simulink model "Commande"  (R2020b)
settings: Solver=VariableStepAuto  StartTime=0.0  StopTime=1  RelTol=1e-3
undefined symbols (not defined in the file or in its folder): FC, FuelCellLoadFcn, gcbh, ln, sps_rtmsupport, Ts
libraries: simulink x43, powerlib x37, powerlib_meascontrol x7, fuzblock x4, powerlib_extras x2
(part 1 of 3)
settings Model: Creator=Abdelhak_Samir  LastModifiedBy=Abdelhak_Samir
settings SolverCC: ZeroCrossAlgorithm=Adaptive
settings DebuggingCC: IgnoredZcDiagnostic=none  UnconnectedInputMsg=none  UnconnectedOutputMsg=none  UnconnectedLineMsg=none
settings ModelReferenceCC: EnableRefExpFcnMdlSchedulingChecks=off
settings RTWCC: GPUComputeCapability=5.0
settings ConfigComp: CovBoundaryAbsTol=1.0e-5

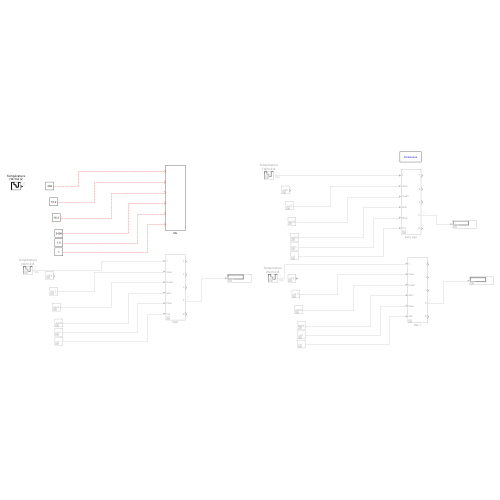
[thumbnail: Simulink's stored preview of the top-level diagram]
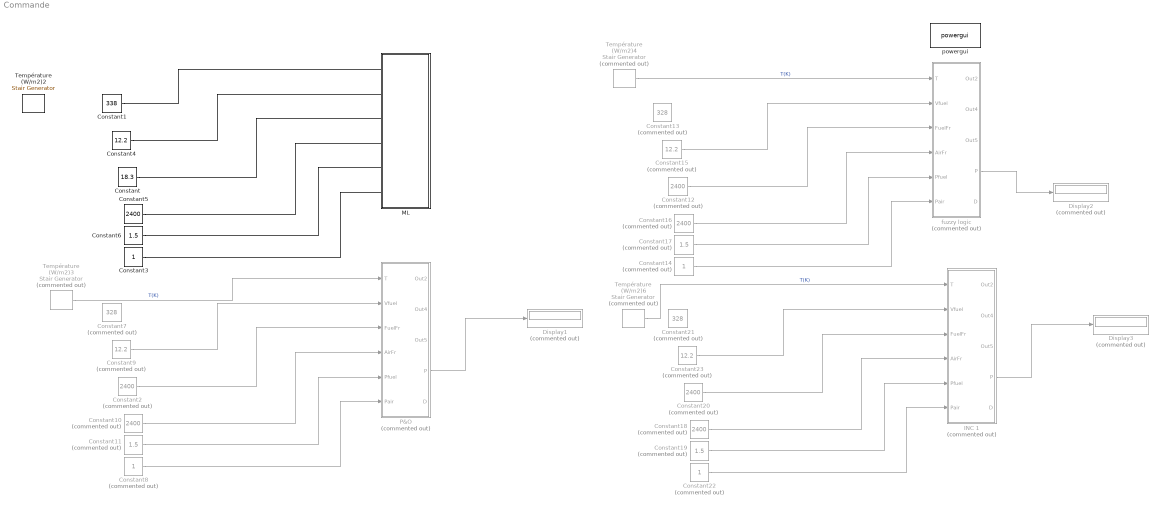
== system Commande ==
  Constant : Constant  Value=18.3
  Constant1 : Constant  Value=338
  Constant{2,10,12,16,18,20} (6 alike) : Constant  Commented=on  Value=2400
  Constant11 : Constant  Commented=on  Value=1.5
  Constant13 : Constant  Commented=on  Value=328
  Constant14 : Constant  Commented=on
  Constant15 : Constant  Commented=on  Value=12.2
  Constant17 : Constant  Commented=on  Value=1.5
  Constant19 : Constant  Commented=on  Value=1.5
  Constant21 : Constant  Commented=on  Value=328
  Constant22 : Constant  Commented=on
  Constant23 : Constant  Commented=on  Value=12.2
  Constant3 : Constant
  Constant4 : Constant  Value=12.2
  Constant5 : Constant  Value=2400
  Constant6 : Constant  Value=1.5
  Constant7 : Constant  Commented=on  Value=328
  Constant8 : Constant  Commented=on
  Constant9 : Constant  Commented=on  Value=12.2
  Display1 : Display  Commented=on
  Display2 : Display  Commented=on
  Display3 : Display  Commented=on
  INC 1 : Subsystem  Commented=on
  ML : Subsystem
  P&O : Subsystem  Commented=on
  Température (W/m2)2 : powerlib_meascontrol/Pulse & Signal Generators/Stair Generator  t=[0, 0.2 , 0.4 , 0.6, 0.8,1]  e=[300,330,320,310,330,330]  Ts=0.00001
  Température (W/m2)3 : powerlib_meascontrol/Pulse & Signal Generators/Stair Generator  Commented=on  t=[0, 0.2 , 0.4 , 0.6, 0.8,1]  e=[300,330,320,310,330,330]  Ts=0.00001
  Température (W/m2)4 : powerlib_meascontrol/Pulse & Signal Generators/Stair Generator  Commented=on  t=[0, 0.2 , 0.4 , 0.6, 0.8,1]  e=[300,330,320,310,330,330]  Ts=0.00001
  Température (W/m2)6 : powerlib_meascontrol/Pulse & Signal Generators/Stair Generator  Commented=on  t=[0, 0.2 , 0.4 , 0.6, 0.8,1]  e=[300,330,320,310,330,330]  Ts=0.00001
  fuzzy logic : Subsystem  Commented=on
  powergui : powerlib/powergui  Priority=1  SimulationMode=Continuous  SampleTime=0.0001  frequency=60  Iterations=50  frequencyindice=0  Pbase=100e6  ErrMax=1e-4  UnitsV=kV  UnitsW=MW  buscounter=0  FunctionMessages=off  echomessages=off  EnableUseOfTLC=off  CurrentSourceSwitches=off  DisableSnubberDevices=off  DisableRonSwitches=off  DisableVfSwitches=off  DisplayEquations=off  AutomaticDiscreteSolvers=off  SolverType=Tustin/Backward Euler (TBE)  Interpol=off  ExternalGateDelay=off  methode=off  Ts=100  x0status=blocks  SPID=on  SwTol=0  HookPort=off  NonlinearTolerance=1e-4  nMaxIteration=100  ContinueOnMaxIteration=off  RestoreLinks=warning  ResistiveCurrentMeasurement=off  Frange=[0:2:500]  Ylog=off  Xlog=on  ShowGrid=off  save=off  variable=ZData  structure=0  ZoomFFT=off  StartTime=0.0  cycles=1  DisplayStyle=1  fundamental=60  FreqAxis=off  MaxFrequency=1000  frequencyindicesteady=1  RmsSteady=1  display=off
  wires:
  Constant4/1 -> ?
  Constant/1 -> ?
  Constant5/1 -> ?
  Constant6/1 -> ?
  Constant3/1 -> ?
  Constant8/1 -> P&O/6(Pair)
  Constant2/1 -> P&O/3(FuelFr)
  Constant9/1 -> P&O/2(Vfuel)
  Constant10/1 -> P&O/4(AirFr)
  P&O/4(P) -> Display1/1
  Constant11/1 -> P&O/5(Pfuel)
  Constant14/1 -> fuzzy logic/6(Pair)
  Constant12/1 -> fuzzy logic/3(FuelFr)
  Constant15/1 -> fuzzy logic/2(Vfuel)
  Constant16/1 -> fuzzy logic/4(AirFr)
  fuzzy logic/4(P) -> Display2/1
  Constant17/1 -> fuzzy logic/5(Pfuel)
  INC 1/4(P) -> Display3/1
  Constant18/1 -> INC 1/4(AirFr)
  Constant20/1 -> INC 1/3(FuelFr)
  Constant22/1 -> INC 1/6(Pair)
  Constant23/1 -> INC 1/2(Vfuel)
  Constant19/1 -> INC 1/5(Pfuel)
  Température (W/m2)4/1 -> fuzzy logic/1(T)  "T(K)"
  Température (W/m2)3/1 -> P&O/1(T)  "T(K)"
  Température (W/m2)6/1 -> INC 1/1(T)  "T(K)"
  Constant1/1 -> ?

== system Commande/INC 1 ==
  note: LOAD
  note: Boost Convertor
  note: Voltage Sensor
  T : Inport
  Vfuel : Inport  Port=2
  FuelFr : Inport  Port=3
  AirFr : Inport  Port=4
  Pfuel : Inport  Port=5
  Pair : Inport  Port=6
  Current Measurement : powerlib/Measurements/Current Measurement  PhasorSimulation=off  OutputType=Complex  PSBequivalent=0
  Demux : Demux  Outputs=5
  Diode : powerlib/Power Electronics/Diode  Ron=0.001  Lon=0  Vf=0.7  IC=0  UseSnubber=0  Rs=500  Cs=250e-9  Measurements=off
  Diode1 : powerlib/Power Electronics/Diode  Ron=0.001  Lon=0  Vf=0.7  IC=0  UseSnubber=0  Rs=500  Cs=250e-9  Measurements=off
  E1 : Product  Inputs=**
  Fuel Cell Stack : Subsystem  AncestorBlock=sps_lib/Sources/Fuel Cell Stack  DialogController=POWERSYS.PowerSysDialog  LoadFcn=sps_rtmsupport('LoadFcn',gcbh);FuelCellLoadFcn(gcb)  StartFcn=sps_rtmsupport('StartFcn',gcbh);  StopFcn=sps_rtmsupport('StopFcn',gcbh);  mask(Fuel Cell Stack){PresetModel=PEMFC - 1.26 kW - 24 Vdc, FcType=0, Detailed=Detailed, Eoc=[42,35], NomVI=[52,24.23], EndVI=[100,20], Nc=42, n=46, TOp=55, AirFr=2400, SuppPress=[1.5,1], Comp=[99.95,21,1], SignX=off, SignY=off, FlowRateH2=on, FlowRateAir=on, SystemTemp=on, SystemPH2=off, SystemPAir=off, FCDyn=off, FC_tau=1, Peak_O2=80, V_Under=10}
      mask prompts: PresetModel "Preset model:"; FcType "Fuel Cell type:"; Detailed "Model detail Level:"; Eoc "Voltage at 0A and 1A [V_0(V), V_1(V)]"; NomVI "Nominal operating point [Inom(A), Vnom(V)]"; EndVI "Maximum operating point [Iend(A), Vend(V)]"; Nc "Number of cells"; n "Nominal stack efficiency (%)"; TOp "Operating temperature (Celsius)"; AirFr "Nominal Air flow rate (lpm)"; SuppPress "Nominal supply pressure [Fuel (bar), Air (bar)]"; Comp "Nominal composition (%) [H2 O2 H2O(Air)]"; SignX "Fuel  composition [x_H2(%)]"; SignY "Oxidant composition [y_O2(%)]"; FlowRateH2 "Fuel flow rate [FuelFr(lpm)]"; FlowRateAir "Air flow rate [AirFr(lpm)]"; SystemTemp "System Temperature [T(Kelvin)]"; SystemPH2 "Fuel supply pressure [Pfuel(bar)]"; SystemPAir "Air supply pressure [PAir(bar)]"; FCDyn "Specify Fuel Cell Dynamics?"; FC_tau "Fuel Cell response time (sec)"; Peak_O2 "Peak O2 utilization (%)"; V_Under "Voltage undershoot (V) @ peak O2 utilization"
      mask help:
      | Implements a generic hydrogen fuel cell model which allows the simulation for the following types of cells:
      | - Proton Exchange Membrane Fuel Cell (PEMFC)
      | - Solid Oxide Fuel Cell (SOFC)
      | - Alkaline Fuel Cell (AFC)
      mask init:
      | block = gcb;
      | %% DO NOT CHANGE THIS ORDER
      | FuelCellCback(block,'Inputs')
      | [FC, WantBlockChoice, Ts] = FuelCellInit(block,Eoc,NomVI,EndVI,Nc,n,TOp,AirFr,SuppPress,Comp,FlowRateH2,FlowRateAir);
      | powericon('SetInternalModels','set',block,WantBlockChoice);
      settings: CopyFcn=sps_rtmsupport('CopyFcn',gcbh);  DeleteFcn=sps_rtmsupport('DeleteFcn',gcbh);  UndoDeleteFcn=sps_rtmsupport('UndoDeleteFcn',gcbh);  ModelCloseFcn=sps_rtmsupport('ModelCloseFcn',gcbh);  PreSaveFcn=sps_rtmsupport('PreSaveFcn',gcbh);  PostSaveFcn=sps_rtmsupport('PostSaveFcn',gcbh);  NameChangeFcn=sps_rtmsupport('NameChangeFcn',gcbh);  PreCopyFcn=sps_rtmsupport('PreCopyFcn',gcbh);  OpenFcn=sps_rtmsupport('OpenFcn',gcbh, [1 2 3 13 14 15 16 17 18 19 20]);  CloseFcn=sps_rtmsupport('CloseFcn',gcbh);  PreDeleteFcn=sps_rtmsupport('PreDeleteFcn',gcbh);
      mask Help: helpview(psbhelp)
      mask TypeOptions PresetModel: No (User-Defined) | PEMFC - 1.26 kW - 24 Vdc | PEMFC - 6 kW - 45 Vdc | PEMFC - 50 kW - 625 Vdc | AFC - 2.4 kW - 48 Vdc | SOFC - 3 kW - 100 Vdc | SOFC - 25 kW - 630 Vdc
      mask Callback PresetModel: FuelCellCback(gcb,'Preset')
      mask TypeOptions Detailed: Simplified | Detailed
      mask Callback Detailed: FuelCellCback(gcb,'Visibilities')
      mask Callback FlowRateAir: FuelCellCback(gcb,'Visibilities')
      mask Callback FCDyn: FuelCellCback(gcb,'Visibilities')
      mask DialogControl ParameterTabVar0 Prompt: Parameters
      mask DialogControl plot_graph Prompt: Plot V_I characteristic
      mask DialogControl plot_graph Callback: FuelCellCback(gcb,'PlotGraph');
      mask DialogControl ViewParam Prompt: View Cell parameters
      mask DialogControl ViewParam Callback: FuelCellCback(gcb,'ViewParam');
      mask DialogControl ParameterTabVar01 Prompt: Signal variation
      mask DialogControl ParameterTabVar012 Prompt: Fuel Cell Dynamics
  Fuzzy Controller : Subsystem  Commented=on
  INC based MPPT : Subsystem
  Mosfet : powerlib/Power Electronics/Mosfet  Ron=0.1  Lon=0  Rd=0.01  Vfd=0.7  IC=0  Rs=1e5  Cs=10^-9  Measurements=off
  PWM Generator (DC-DC)1 : powerlib_meascontrol/Pulse & Signal Generators/PWM Generator (DC-DC)  Fsw=10000  Ts=0
  Pn : Product
  Scope : Scope  NumInputPorts=2
  Scope1 : Scope
  Scope2 : Scope
  Series RLC Branch : powerlib/Elements/Series RLC Branch  LConnTagsString=__new0  RConnTagsString=__new0  BranchType=L  Resistance=1  Inductance=1e-4  SetiL0=off  InitialCurrent=0  Capacitance=1e-6  Setx0=off  InitialVoltage=0  Measurements=None
  Series RLC Branch1 : powerlib/Elements/Series RLC Branch  LConnTagsString=__new0  RConnTagsString=__new0  BranchType=C  Resistance=1  Inductance=1e-4  SetiL0=off  InitialCurrent=0  Capacitance=4700e-6  Setx0=off  InitialVoltage=0  Measurements=None
  Series RLC Branch4 : powerlib/Elements/Series RLC Branch  LConnTagsString=__new0  RConnTagsString=__new0  BranchType=C  Resistance=1  Inductance=1e-4  SetiL0=off  InitialCurrent=0  Capacitance=4700e-5  Setx0=on  InitialVoltage=42  Measurements=None
  Series RLC Load1 : powerlib/Elements/Series RLC Load  LConnTagsString=a  RConnTagsString=__new0  NominalVoltage=50  NominalFrequency=500  ActivePower=33  InductivePower=0  CapacitivePower=0  Setx0=off  InitialVoltage=0  SetiL0=off  InitialCurrent=0  Measurements=None  LoadType=constant Z
  Voltage Measurement1 : powerlib/Measurements/Voltage Measurement  PhasorSimulation=off  OutputType=Complex  PSBequivalent=0
  Out2 : Outport
  Out4 : Outport  Port=2
  Out5 : Outport  Port=3
  P : Outport  Port=4
  D : Outport  Port=5
  wires:
  Current Measurement/1 -> E1/1  "Iout"
  Pn/1 -> P/1, Scope/2, Fuzzy Controller/2(P), Scope1/1  "P"
  PWM Generator (DC-DC)1/1 -> Mosfet/1
  Demux/1 -> Fuzzy Controller/1(Vin), INC based MPPT/1(Vpv), Scope2/1, Pn/1  "Vin"
  Fuzzy Controller/1(D) -> D/1
  Demux/5 -> Out5/1
  Demux/2 -> INC based MPPT/2(Ipv), Pn/2  "Iin"
  FuelFr/1 -> Fuel Cell Stack/1(FuelFr)
  Fuel Cell Stack/1(m) -> Demux/1
  E1/1 -> Scope/1  "Pout"
  AirFr/1 -> Fuel Cell Stack/2(AirFr)
  Voltage Measurement1/1 -> E1/2  "Vout"
  INC based MPPT/1(PWM1) -> PWM Generator (DC-DC)1/1
  Demux/3 -> Out2/1
  Demux/4 -> Out4/1
  T/1 -> Fuel Cell Stack/3(T)
  connections:
  Series RLC Branch4/LConn1 -- Series RLC Branch/LConn1 -- Diode1/RConn1
  Series RLC Branch1/LConn1 -- Diode/RConn1 -- Current Measurement/LConn1
  Fuel Cell Stack/RConn1 -- Diode1/LConn1
  Mosfet/RConn1 -- Fuel Cell Stack/RConn2 -- Series RLC Branch4/RConn1 -- Voltage Measurement1/LConn2 -- Series RLC Load1/RConn1 -- Series RLC Branch1/RConn1
  Current Measurement/RConn1 -- Series RLC Load1/LConn1 -- Voltage Measurement1/LConn1
  Mosfet/LConn1 -- Diode/LConn1 -- Series RLC Branch/RConn1

== system Commande/ML ==
  ML Model : Subsystem

== system Commande/P&O ==
  note: LOAD
  note: Boost Convertor
  note: Voltage Sensor
  T : Inport
  Vfuel : Inport  Port=2
  FuelFr : Inport  Port=3
  AirFr : Inport  Port=4
  Pfuel : Inport  Port=5
  Pair : Inport  Port=6
  Current Measurement : powerlib/Measurements/Current Measurement  PhasorSimulation=off  OutputType=Complex  PSBequivalent=0
  Demux : Demux  Outputs=5
  Diode : powerlib/Power Electronics/Diode  Ron=0.001  Lon=0  Vf=0.7  IC=0  UseSnubber=0  Rs=500  Cs=250e-9  Measurements=off
  Diode1 : powerlib/Power Electronics/Diode  Ron=0.001  Lon=0  Vf=0.7  IC=0  UseSnubber=0  Rs=500  Cs=250e-9  Measurements=off
  E1 : Product  Inputs=**
  Fuel Cell Stack : Subsystem  AncestorBlock=sps_lib/Sources/Fuel Cell Stack  DialogController=POWERSYS.PowerSysDialog  LoadFcn=sps_rtmsupport('LoadFcn',gcbh);FuelCellLoadFcn(gcb)  StartFcn=sps_rtmsupport('StartFcn',gcbh);  StopFcn=sps_rtmsupport('StopFcn',gcbh);  mask(Fuel Cell Stack){PresetModel=PEMFC - 1.26 kW - 24 Vdc, FcType=0, Detailed=Detailed, Eoc=[42,35], NomVI=[52,24.23], EndVI=[100,20], Nc=42, n=46, TOp=55, AirFr=2400, SuppPress=[1.5,1], Comp=[99.95,21,1], SignX=off, SignY=off, FlowRateH2=on, FlowRateAir=on, SystemTemp=on, SystemPH2=off, SystemPAir=off, FCDyn=off, FC_tau=1, Peak_O2=80, V_Under=10}
      mask prompts: PresetModel "Preset model:"; FcType "Fuel Cell type:"; Detailed "Model detail Level:"; Eoc "Voltage at 0A and 1A [V_0(V), V_1(V)]"; NomVI "Nominal operating point [Inom(A), Vnom(V)]"; EndVI "Maximum operating point [Iend(A), Vend(V)]"; Nc "Number of cells"; n "Nominal stack efficiency (%)"; TOp "Operating temperature (Celsius)"; AirFr "Nominal Air flow rate (lpm)"; SuppPress "Nominal supply pressure [Fuel (bar), Air (bar)]"; Comp "Nominal composition (%) [H2 O2 H2O(Air)]"; SignX "Fuel  composition [x_H2(%)]"; SignY "Oxidant composition [y_O2(%)]"; FlowRateH2 "Fuel flow rate [FuelFr(lpm)]"; FlowRateAir "Air flow rate [AirFr(lpm)]"; SystemTemp "System Temperature [T(Kelvin)]"; SystemPH2 "Fuel supply pressure [Pfuel(bar)]"; SystemPAir "Air supply pressure [PAir(bar)]"; FCDyn "Specify Fuel Cell Dynamics?"; FC_tau "Fuel Cell response time (sec)"; Peak_O2 "Peak O2 utilization (%)"; V_Under "Voltage undershoot (V) @ peak O2 utilization"
      mask help:
      | Implements a generic hydrogen fuel cell model which allows the simulation for the following types of cells:
      | - Proton Exchange Membrane Fuel Cell (PEMFC)
      | - Solid Oxide Fuel Cell (SOFC)
      | - Alkaline Fuel Cell (AFC)
      mask init: same as Commande/INC 1/Fuel Cell Stack
      settings: CopyFcn=sps_rtmsupport('CopyFcn',gcbh);  DeleteFcn=sps_rtmsupport('DeleteFcn',gcbh);  UndoDeleteFcn=sps_rtmsupport('UndoDeleteFcn',gcbh);  ModelCloseFcn=sps_rtmsupport('ModelCloseFcn',gcbh);  PreSaveFcn=sps_rtmsupport('PreSaveFcn',gcbh);  PostSaveFcn=sps_rtmsupport('PostSaveFcn',gcbh);  NameChangeFcn=sps_rtmsupport('NameChangeFcn',gcbh);  PreCopyFcn=sps_rtmsupport('PreCopyFcn',gcbh);  OpenFcn=sps_rtmsupport('OpenFcn',gcbh, [1 2 3 13 14 15 16 17 18 19 20]);  CloseFcn=sps_rtmsupport('CloseFcn',gcbh);  PreDeleteFcn=sps_rtmsupport('PreDeleteFcn',gcbh);
      mask Help: helpview(psbhelp)
      mask TypeOptions PresetModel: No (User-Defined) | PEMFC - 1.26 kW - 24 Vdc | PEMFC - 6 kW - 45 Vdc | PEMFC - 50 kW - 625 Vdc | AFC - 2.4 kW - 48 Vdc | SOFC - 3 kW - 100 Vdc | SOFC - 25 kW - 630 Vdc
      mask Callback PresetModel: FuelCellCback(gcb,'Preset')
      mask TypeOptions Detailed: Simplified | Detailed
      mask Callback Detailed: FuelCellCback(gcb,'Visibilities')
      mask Callback FlowRateAir: FuelCellCback(gcb,'Visibilities')
      mask Callback FCDyn: FuelCellCback(gcb,'Visibilities')
      mask DialogControl ParameterTabVar0 Prompt: Parameters
      mask DialogControl plot_graph Prompt: Plot V_I characteristic
      mask DialogControl plot_graph Callback: FuelCellCback(gcb,'PlotGraph');
      mask DialogControl ViewParam Prompt: View Cell parameters
      mask DialogControl ViewParam Callback: FuelCellCback(gcb,'ViewParam');
      mask DialogControl ParameterTabVar01 Prompt: Signal variation
      mask DialogControl ParameterTabVar012 Prompt: Fuel Cell Dynamics
  Fuzzy Controller : Subsystem  Commented=on
  Mosfet : powerlib/Power Electronics/Mosfet  Ron=0.1  Lon=0  Rd=0.01  Vfd=0.7  IC=0  Rs=1e5  Cs=10^-9  Measurements=off
  P&O base MPPT : Subsystem
  PWM Generator (DC-DC)1 : powerlib_meascontrol/Pulse & Signal Generators/PWM Generator (DC-DC)  Fsw=10000  Ts=0
  Pn : Product
  Scope : Scope  NumInputPorts=2
  Scope1 : Scope
  Scope2 : Scope
  Series RLC Branch : powerlib/Elements/Series RLC Branch  LConnTagsString=__new0  RConnTagsString=__new0  BranchType=L  Resistance=1  Inductance=1e-4  SetiL0=off  InitialCurrent=0  Capacitance=1e-6  Setx0=off  InitialVoltage=0  Measurements=None
  Series RLC Branch1 : powerlib/Elements/Series RLC Branch  LConnTagsString=__new0  RConnTagsString=__new0  BranchType=C  Resistance=1  Inductance=1e-4  SetiL0=off  InitialCurrent=0  Capacitance=4700e-6  Setx0=off  InitialVoltage=0  Measurements=None
  Series RLC Branch4 : powerlib/Elements/Series RLC Branch  LConnTagsString=__new0  RConnTagsString=__new0  BranchType=C  Resistance=1  Inductance=1e-4  SetiL0=off  InitialCurrent=0  Capacitance=4700e-5  Setx0=on  InitialVoltage=42  Measurements=None
  Series RLC Load1 : powerlib/Elements/Series RLC Load  LConnTagsString=a  RConnTagsString=__new0  NominalVoltage=50  NominalFrequency=500  ActivePower=33  InductivePower=0  CapacitivePower=0  Setx0=off  InitialVoltage=0  SetiL0=off  InitialCurrent=0  Measurements=None  LoadType=constant Z
  Voltage Measurement1 : powerlib/Measurements/Voltage Measurement  PhasorSimulation=off  OutputType=Complex  PSBequivalent=0
  Out2 : Outport
  Out4 : Outport  Port=2
  Out5 : Outport  Port=3
  P : Outport  Port=4
  D : Outport  Port=5
  wires:
  Current Measurement/1 -> E1/1  "Iout"
  Pn/1 -> P/1, Scope/2, Fuzzy Controller/2(P), Scope1/1  "P"
  PWM Generator (DC-DC)1/1 -> Mosfet/1
  Demux/1 -> Scope2/1, Fuzzy Controller/1(Vin), P&O base MPPT/1(Vpv), Pn/1  "Vin"
  Fuzzy Controller/1(D) -> D/1
  Demux/5 -> Out5/1
  Demux/2 -> P&O base MPPT/2(Ipv), Pn/2  "Iin"
  FuelFr/1 -> Fuel Cell Stack/1(FuelFr)
  Fuel Cell Stack/1(m) -> Demux/1
  E1/1 -> Scope/1  "Pout"
  AirFr/1 -> Fuel Cell Stack/2(AirFr)
  Voltage Measurement1/1 -> E1/2  "Vout"
  P&O base MPPT/1(PWM) -> PWM Generator (DC-DC)1/1
  Demux/3 -> Out2/1
  Demux/4 -> Out4/1
  T/1 -> Fuel Cell Stack/3(T)
  connections:
  Series RLC Branch4/LConn1 -- Series RLC Branch/LConn1 -- Diode1/RConn1
  Series RLC Branch1/LConn1 -- Diode/RConn1 -- Current Measurement/LConn1
  Fuel Cell Stack/RConn1 -- Diode1/LConn1
  Mosfet/RConn1 -- Fuel Cell Stack/RConn2 -- Series RLC Branch4/RConn1 -- Voltage Measurement1/LConn2 -- Series RLC Load1/RConn1 -- Series RLC Branch1/RConn1
  Current Measurement/RConn1 -- Series RLC Load1/LConn1 -- Voltage Measurement1/LConn1
  Mosfet/LConn1 -- Diode/LConn1 -- Series RLC Branch/RConn1

== system Commande/fuzzy logic ==
  note: LOAD
  note: Boost Convertor
  note: Voltage Sensor
  T : Inport
  Vfuel : Inport  Port=2
  FuelFr : Inport  Port=3
  AirFr : Inport  Port=4
  Pfuel : Inport  Port=5
  Pair : Inport  Port=6
  Constant : Constant  Value=330
  Current Measurement : powerlib/Measurements/Current Measurement  PhasorSimulation=off  OutputType=Complex  PSBequivalent=0
  Demux : Demux  Outputs=5
  Diode : powerlib/Power Electronics/Diode  Ron=0.001  Lon=0  Vf=0.7  IC=0  UseSnubber=0  Rs=500  Cs=250e-9  Measurements=off
  Diode1 : powerlib/Power Electronics/Diode  Ron=0.001  Lon=0  Vf=0.7  IC=0  UseSnubber=0  Rs=500  Cs=250e-9  Measurements=off
  Display : Display
  E1 : Product  Inputs=**
  Fuel Cell Stack1 : Subsystem  AncestorBlock=sps_lib/Sources/Fuel Cell Stack  DialogController=POWERSYS.PowerSysDialog  LoadFcn=sps_rtmsupport('LoadFcn',gcbh);FuelCellLoadFcn(gcb)  StartFcn=sps_rtmsupport('StartFcn',gcbh);  StopFcn=sps_rtmsupport('StopFcn',gcbh);  mask(Fuel Cell Stack){PresetModel=PEMFC - 1.26 kW - 24 Vdc, FcType=0, Detailed=Detailed, Eoc=[42,35], NomVI=[52,24.23], EndVI=[100,20], Nc=42, n=46, TOp=55, AirFr=2400, SuppPress=[1.5,1], Comp=[99.95,21,1], SignX=off, SignY=off, FlowRateH2=on, FlowRateAir=on, SystemTemp=on, SystemPH2=off, SystemPAir=off, FCDyn=off, FC_tau=1, Peak_O2=80, V_Under=10}
      mask prompts: PresetModel "Preset model:"; FcType "Fuel Cell type:"; Detailed "Model detail Level:"; Eoc "Voltage at 0A and 1A [V_0(V), V_1(V)]"; NomVI "Nominal operating point [Inom(A), Vnom(V)]"; EndVI "Maximum operating point [Iend(A), Vend(V)]"; Nc "Number of cells"; n "Nominal stack efficiency (%)"; TOp "Operating temperature (Celsius)"; AirFr "Nominal Air flow rate (lpm)"; SuppPress "Nominal supply pressure [Fuel (bar), Air (bar)]"; Comp "Nominal composition (%) [H2 O2 H2O(Air)]"; SignX "Fuel  composition [x_H2(%)]"; SignY "Oxidant composition [y_O2(%)]"; FlowRateH2 "Fuel flow rate [FuelFr(lpm)]"; FlowRateAir "Air flow rate [AirFr(lpm)]"; SystemTemp "System Temperature [T(Kelvin)]"; SystemPH2 "Fuel supply pressure [Pfuel(bar)]"; SystemPAir "Air supply pressure [PAir(bar)]"; FCDyn "Specify Fuel Cell Dynamics?"; FC_tau "Fuel Cell response time (sec)"; Peak_O2 "Peak O2 utilization (%)"; V_Under "Voltage undershoot (V) @ peak O2 utilization"
      mask help:
      | Implements a generic hydrogen fuel cell model which allows the simulation for the following types of cells:
      | - Proton Exchange Membrane Fuel Cell (PEMFC)
      | - Solid Oxide Fuel Cell (SOFC)
      | - Alkaline Fuel Cell (AFC)
      mask init: same as Commande/INC 1/Fuel Cell Stack
      settings: CopyFcn=sps_rtmsupport('CopyFcn',gcbh);  DeleteFcn=sps_rtmsupport('DeleteFcn',gcbh);  UndoDeleteFcn=sps_rtmsupport('UndoDeleteFcn',gcbh);  ModelCloseFcn=sps_rtmsupport('ModelCloseFcn',gcbh);  PreSaveFcn=sps_rtmsupport('PreSaveFcn',gcbh);  PostSaveFcn=sps_rtmsupport('PostSaveFcn',gcbh);  NameChangeFcn=sps_rtmsupport('NameChangeFcn',gcbh);  PreCopyFcn=sps_rtmsupport('PreCopyFcn',gcbh);  OpenFcn=sps_rtmsupport('OpenFcn',gcbh, [1 2 3 13 14 15 16 17 18 19 20]);  CloseFcn=sps_rtmsupport('CloseFcn',gcbh);  PreDeleteFcn=sps_rtmsupport('PreDeleteFcn',gcbh);
      mask Help: helpview(psbhelp)
      mask TypeOptions PresetModel: No (User-Defined) | PEMFC - 1.26 kW - 24 Vdc | PEMFC - 6 kW - 45 Vdc | PEMFC - 50 kW - 625 Vdc | AFC - 2.4 kW - 48 Vdc | SOFC - 3 kW - 100 Vdc | SOFC - 25 kW - 630 Vdc
      mask Callback PresetModel: FuelCellCback(gcb,'Preset')
      mask TypeOptions Detailed: Simplified | Detailed
      mask Callback Detailed: FuelCellCback(gcb,'Visibilities')
      mask Callback FlowRateAir: FuelCellCback(gcb,'Visibilities')
      mask Callback FCDyn: FuelCellCback(gcb,'Visibilities')
      mask DialogControl ParameterTabVar0 Prompt: Parameters
      mask DialogControl plot_graph Prompt: Plot V_I characteristic
      mask DialogControl plot_graph Callback: FuelCellCback(gcb,'PlotGraph');
      mask DialogControl ViewParam Prompt: View Cell parameters
      mask DialogControl ViewParam Callback: FuelCellCback(gcb,'ViewParam');
      mask DialogControl ParameterTabVar01 Prompt: Signal variation
      mask DialogControl ParameterTabVar012 Prompt: Fuel Cell Dynamics
  Fuzzy Controller : Subsystem  Commented=on
  Fuzzy Controller2 : Subsystem
  Mosfet : powerlib/Power Electronics/Mosfet  Ron=0.1  Lon=0  Rd=0.01  Vfd=0.7  IC=0  Rs=1e5  Cs=10^-9  Measurements=off
  PWM Generator (DC-DC) : powerlib_meascontrol/Pulse & Signal Generators/PWM Generator (DC-DC)  Fsw=10000  Ts=0
  Pn : Product
  Scope : Scope  NumInputPorts=2
  Series RLC Branch : powerlib/Elements/Series RLC Branch  LConnTagsString=__new0  RConnTagsString=__new0  BranchType=L  Resistance=1  Inductance=1e-4  SetiL0=off  InitialCurrent=0  Capacitance=1e-6  Setx0=off  InitialVoltage=0  Measurements=None
  Series RLC Branch1 : powerlib/Elements/Series RLC Branch  LConnTagsString=__new0  RConnTagsString=__new0  BranchType=C  Resistance=1  Inductance=1e-4  SetiL0=off  InitialCurrent=0  Capacitance=4700e-6  Setx0=off  InitialVoltage=0  Measurements=None
  Series RLC Branch4 : powerlib/Elements/Series RLC Branch  LConnTagsString=__new0  RConnTagsString=__new0  BranchType=C  Resistance=1  Inductance=1e-4  SetiL0=off  InitialCurrent=0  Capacitance=4700e-5  Setx0=on  InitialVoltage=42  Measurements=None
  Series RLC Load1 : powerlib/Elements/Series RLC Load  LConnTagsString=a  RConnTagsString=__new0  NominalVoltage=50  NominalFrequency=500  ActivePower=33  InductivePower=0  CapacitivePower=0  Setx0=off  InitialVoltage=0  SetiL0=off  InitialCurrent=0  Measurements=None  LoadType=constant Z
  Voltage Measurement1 : powerlib/Measurements/Voltage Measurement  PhasorSimulation=off  OutputType=Complex  PSBequivalent=0
  Out2 : Outport
  Out4 : Outport  Port=2
  Out5 : Outport  Port=3
  P : Outport  Port=4
  D : Outport  Port=5
  wires:
  Current Measurement/1 -> E1/1  "Iout"
  Pn/1 -> Fuzzy Controller2/2(P), Display/1, P/1, Scope/2, Fuzzy Controller/2(P)  "P"
  Demux/1 -> Fuzzy Controller2/1(Vin), Fuzzy Controller/1(Vin), Pn/1  "Vin"
  Fuzzy Controller/1(D) -> D/1
  Demux/5 -> Out5/1
  Demux/2 -> Pn/2  "Iin"
  Fuel Cell Stack1/1(m) -> Demux/1
  E1/1 -> Scope/1  "Pout"
  Voltage Measurement1/1 -> E1/2  "Vout"
  PWM Generator (DC-DC)/1 -> Mosfet/1
  Demux/3 -> Out2/1
  Demux/4 -> Out4/1
  Fuzzy Controller2/1(D) -> PWM Generator (DC-DC)/1
  AirFr/1 -> Fuel Cell Stack1/2(AirFr)
  FuelFr/1 -> Fuel Cell Stack1/1(FuelFr)
  T/1 -> Fuel Cell Stack1/3(T)
  connections:
  Series RLC Branch4/LConn1 -- Series RLC Branch/LConn1 -- Diode1/RConn1
  Series RLC Branch1/LConn1 -- Diode/RConn1 -- Current Measurement/LConn1
  Fuel Cell Stack1/RConn1 -- Diode1/LConn1
  Mosfet/RConn1 -- Fuel Cell Stack1/RConn2 -- Series RLC Branch4/RConn1 -- Series RLC Load1/RConn1 -- Voltage Measurement1/LConn2 -- Series RLC Branch1/RConn1
  Current Measurement/RConn1 -- Voltage Measurement1/LConn1 -- Series RLC Load1/LConn1
  Mosfet/LConn1 -- Diode/LConn1 -- Series RLC Branch/RConn1

== system Commande/INC 1/Fuel Cell Stack ==
  FuelFr : Inport
  AirFr : Inport  Port=2
  T : Inport  Port=3
  Controlled Voltage Source1 : powerlib/Electrical Sources/Controlled Voltage Source  Initialize=on  Source_Type=AC  Amplitude=0  Phase=0  Frequency=0  Measurements=None
  Current Measurement1 : powerlib/Measurements/Current Measurement  PhasorSimulation=off  OutputType=Complex  PSBequivalent=0
  Diode1 : powerlib/Power Electronics/Diode  Ron=FC.Rohm  Lon=0  Vf=0  IC=0  UseSnubber=off  Rs=1e4  Cs=inf  Measurements=off
  Gain1 : Gain  Gain=0.01
  Gain3 : Gain  Gain=0.01
  Model : Subsystem  AncestorBlock=sps_lib/Sources/Fuel Cell Stack/Model  Variant=on  VariantControlMode=label  LabelModeActiveChoice=Continuous/Detailed
      settings: AttributesFormatString=%<BlockChoice>
  PAir : Constant  Value=FC.PAir
  Pfuel : Constant  Value=FC.Pf
  x_H2 : Constant  Value=FC.x*100
  y_O2 : Constant  Value=FC.y*100
  + : PMIOPort  Tag=PMCPort  Side=Right
  - : PMIOPort  Tag=PMCPort  Port=2  Side=Right
  m : Outport  VectorParamsAs1DForOutWhenUnconnected=off
  wires:
  PAir/1 -> Model/8(PAir)
  Pfuel/1 -> Model/7(Pf)
  T/1 -> Model/2(Op Temp)
  Model/1(Voltage) -> Controlled Voltage Source1/1
  Current Measurement1/1 -> Model/1(Current)
  Model/2(m) -> m/1
  FuelFr/1 -> Model/3(H2)
  x_H2/1 -> Gain1/1
  AirFr/1 -> Model/5(Air)
  y_O2/1 -> Gain3/1
  Gain1/1 -> Model/4(x_H2)
  Gain3/1 -> Model/6(y_O2)
  connections:
  Current Measurement1/LConn1 -- Controlled Voltage Source1/RConn1
  Current Measurement1/RConn1 -- Diode1/LConn1
  -/RConn1 -- Controlled Voltage Source1/LConn1
  Diode1/RConn1 -- +/RConn1

== system Commande/INC 1/Fuzzy Controller ==
  note: DE
  Vin : Inport
  P : Inport  Port=2
  Add : Sum
  DE : Sum  Inputs=+-
  E : Product  Inputs=/*
  Fuzzy Logic Controller with Ruleviewer : fuzblock/Fuzzy Logic  Controller  with Ruleviewer  fismatrix=twnty_five_rules_2  Ts=0.1
  Gain1 : Gain
  Memory1 : Memory  InheritSampleTime=on
  Memory2 : Memory  InheritSampleTime=on
  Memory3 : Memory
  Memory4 : Memory  InheritSampleTime=on
  Mux : Mux  Inputs=2
  Saturation : Saturate  UpperLimit=0.9  LowerLimit=0.1
  Zero-Order Hold : ZeroOrderHold  SampleTime=-1
  Zero-Order Hold1 : ZeroOrderHold  SampleTime=-1
  dP : Sum  Inputs=|+-
  dV : Sum  Inputs=-+
  D : Outport
  wires:
  DE/1 -> Mux/2  "DE"
  Fuzzy Logic Controller with Ruleviewer/1 -> Gain1/1  "DeltaD_Pur"
  Zero-Order Hold/1 -> dP/2, Memory1/1
  dV/1 -> E/1
  dP/1 -> E/2
  E/1 -> DE/1, Memory2/1, Mux/1  "E"
  Mux/1 -> Fuzzy Logic Controller with Ruleviewer/1
  Memory4/1 -> dV/1
  Memory1/1 -> dP/1
  Zero-Order Hold1/1 -> Memory4/1, dV/2
  Gain1/1 -> Add/1  "DeltaD"
  Memory3/1 -> Add/2
  Saturation/1 -> D/1, Memory3/1  "D"
  Memory2/1 -> DE/2
  Add/1 -> Saturation/1
  Vin/1 -> Zero-Order Hold1/1
  P/1 -> Zero-Order Hold/1

== system Commande/INC 1/INC based MPPT ==
  Vpv : Inport
  Ipv : Inport  Port=2
  Add1 : Sum  Inputs=|++
  Add2 : Sum  Inputs=+-
  Add3 : Sum  Inputs=+-
  Add4 : Sum  Inputs=+-
  Compare To Zero : simulink/Logic and Bit Operations/Compare To Zero  relop=~=  OutDataTypeStr=uint8
  Constant2 : Constant  Value=1e-6
  Dead Zone1 : DeadZone  LowerValue=-0.02  UpperValue=+0.02  SaturateOnIntegerOverflow=on
  Gain : Gain
  Initial Duty Cycle1 : Constant  Value=0.5
  Saturation : Saturate  UpperLimit=0.9  LowerLimit=0.1
  Saturation1 : Saturate  UpperLimit=inf  LowerLimit=eps
  Switch2 : Switch  Criteria=u2 ~= 0
  Vb : Memory  InheritSampleTime=on  LinearizeAsDelay=on
  Vb1 : Memory  InheritSampleTime=on  LinearizeAsDelay=on
  div1 : Product  Inputs=*/  RndMeth=Zero
  div2 : Product  Inputs=*/  RndMeth=Zero
  PWM1 : Outport
  wires:
  Add4/1 -> Saturation/1  "D"
  Gain/1 -> Add4/2
  Initial Duty Cycle1/1 -> Add4/1
  Add3/1 -> Compare To Zero/1, Switch2/1  "dV"
  div2/1 -> Add1/2  "I/V"
  Saturation1/1 -> div2/2
  Vb1/1 -> Add3/2
  Add2/1 -> div1/1  "dI"
  Switch2/1 -> div1/2
  Vb/1 -> Add2/2
  Ipv/1 -> Vb/1, Add2/1, div2/1  "I"
  div1/1 -> Add1/1  "dI/dV"
  Compare To Zero/1 -> Switch2/2
  Constant2/1 -> Switch2/3
  Vpv/1 -> Add3/1, Vb1/1, Saturation1/1  "V"
  Add1/1 -> Gain/1  "error"
  Saturation/1 -> PWM1/1

== system Commande/ML/ML Model ==
  Vin : Inport
  T : Inport  Port=2
  Vfuel : Inport  Port=3
  Vout : Inport  Port=4
  Vair : Inport  Port=5
  Pfuel : Inport  Port=6
  Pair : Inport  Port=7
  Constant8 : Constant
  E : Product  Inputs=*/
  Gain : Gain  Gain=1000
  MATLAB Function : MATLAB Function  TreatAsAtomicUnit=on
  Saturation : Saturate  UpperLimit=0.9  LowerLimit=0.1
  Scope3 : Scope
  Sum1 : Sum  Inputs=|+-
  Sum2 : Sum  Inputs=|+-
  D : Outport
  wires:
  Saturation/1 -> D/1, Scope3/1
  Gain/1 -> E/1
  MATLAB Function/1(Vmpp) -> Sum2/1  "Vref"
  Sum1/1 -> Saturation/1  "D"
  Pair/1 -> MATLAB Function/3(Pair)
  Sum2/1 -> Gain/1  "D"
  E/1 -> Sum1/2
  T/1 -> MATLAB Function/1(T)
  Constant8/1 -> Sum1/1
  Vin/1 -> Sum2/2
  Vout/1 -> E/2
  Pfuel/1 -> MATLAB Function/2(Pfuel)
  Vfuel/1 -> MATLAB Function/4(Vfuel)
  Vair/1 -> MATLAB Function/5(Vair)

== system Commande/P&O/Fuel Cell Stack ==
  FuelFr : Inport
  AirFr : Inport  Port=2
  T : Inport  Port=3
  Controlled Voltage Source1 : powerlib/Electrical Sources/Controlled Voltage Source  Initialize=on  Source_Type=AC  Amplitude=0  Phase=0  Frequency=0  Measurements=None
  Current Measurement1 : powerlib/Measurements/Current Measurement  PhasorSimulation=off  OutputType=Complex  PSBequivalent=0
  Diode1 : powerlib/Power Electronics/Diode  Ron=FC.Rohm  Lon=0  Vf=0  IC=0  UseSnubber=off  Rs=1e4  Cs=inf  Measurements=off
  Gain1 : Gain  Gain=0.01
  Gain3 : Gain  Gain=0.01
  Model : Subsystem  AncestorBlock=sps_lib/Sources/Fuel Cell Stack/Model  Variant=on  VariantControlMode=label  LabelModeActiveChoice=Continuous/Detailed
      settings: AttributesFormatString=%<BlockChoice>
  PAir : Constant  Value=FC.PAir
  Pfuel : Constant  Value=FC.Pf
  x_H2 : Constant  Value=FC.x*100
  y_O2 : Constant  Value=FC.y*100
  + : PMIOPort  Tag=PMCPort  Side=Right
  - : PMIOPort  Tag=PMCPort  Port=2  Side=Right
  m : Outport  VectorParamsAs1DForOutWhenUnconnected=off
  wires:
  PAir/1 -> Model/8(PAir)
  Pfuel/1 -> Model/7(Pf)
  T/1 -> Model/2(Op Temp)
  Model/1(Voltage) -> Controlled Voltage Source1/1
  Current Measurement1/1 -> Model/1(Current)
  Model/2(m) -> m/1
  FuelFr/1 -> Model/3(H2)
  x_H2/1 -> Gain1/1
  AirFr/1 -> Model/5(Air)
  y_O2/1 -> Gain3/1
  Gain1/1 -> Model/4(x_H2)
  Gain3/1 -> Model/6(y_O2)
  connections:
  Current Measurement1/LConn1 -- Controlled Voltage Source1/RConn1
  Current Measurement1/RConn1 -- Diode1/LConn1
  -/RConn1 -- Controlled Voltage Source1/LConn1
  Diode1/RConn1 -- +/RConn1

== system Commande/P&O/Fuzzy Controller ==
  note: DE
  Vin : Inport
  P : Inport  Port=2
  Add : Sum
  DE : Sum  Inputs=+-
  E : Product  Inputs=/*
  Fuzzy Logic Controller with Ruleviewer : fuzblock/Fuzzy Logic  Controller  with Ruleviewer  fismatrix=twnty_five_rules_2  Ts=0.1
  Gain1 : Gain
  Memory1 : Memory  InheritSampleTime=on
  Memory2 : Memory  InheritSampleTime=on
  Memory3 : Memory
  Memory4 : Memory  InheritSampleTime=on
  Mux : Mux  Inputs=2
  Saturation : Saturate  UpperLimit=0.9  LowerLimit=0.1
  Zero-Order Hold : ZeroOrderHold  SampleTime=-1
  Zero-Order Hold1 : ZeroOrderHold  SampleTime=-1
  dP : Sum  Inputs=|+-
  dV : Sum  Inputs=-+
  D : Outport
  wires:
  DE/1 -> Mux/2  "DE"
  Fuzzy Logic Controller with Ruleviewer/1 -> Gain1/1  "DeltaD_Pur"
  Zero-Order Hold/1 -> dP/2, Memory1/1
  dV/1 -> E/1
  dP/1 -> E/2
  E/1 -> DE/1, Memory2/1, Mux/1  "E"
  Mux/1 -> Fuzzy Logic Controller with Ruleviewer/1
  Memory4/1 -> dV/1
  Memory1/1 -> dP/1
  Zero-Order Hold1/1 -> Memory4/1, dV/2
  Gain1/1 -> Add/1  "DeltaD"
  Memory3/1 -> Add/2
  Saturation/1 -> D/1, Memory3/1  "D"
  Memory2/1 -> DE/2
  Add/1 -> Saturation/1
  Vin/1 -> Zero-Order Hold1/1
  P/1 -> Zero-Order Hold/1

== system Commande/P&O/P&O base MPPT ==
  note: D
  Vpv : Inport
  Ipv : Inport  Port=2
  D State : Product  RndMeth=Zero
  DeltaD : Constant  Value=0.05
  DeltaP*DeltaV : Product  RndMeth=Zero
  I Filter : powerlib_extras/Control  Blocks/1st-Order  Filter  FilterType=Lowpass  Tc=1e-3  Initialize=off  Vac_Init=[0.8 -25 60]  Vdc_Init=-0.4  PlotResponse=off  param1=[1 500 1]
  Ib : Memory  InheritSampleTime=on  LinearizeAsDelay=on
  If DeltaP*DeltaV<0 : Constant
  If DeltaP*DeltaV>0 : Constant  Value=-1
  Memory2 : Memory  InheritSampleTime=on
  Pb : Product  RndMeth=Zero
  Pn : Product  RndMeth=Zero
  Pn-Pb : Sum  Inputs=+-
  Saturation1 : Saturate  UpperLimit=0.9  LowerLimit=0.1
  Sum : Sum  Inputs=|++
  Switch1 : Switch
  V Filter : powerlib_extras/Control  Blocks/1st-Order  Filter  FilterType=Lowpass  Tc=1e-3  Initialize=off  Vac_Init=[0.8 -25 60]  Vdc_Init=-0.4  PlotResponse=off  param1=[1 500 1]
  Vb : Memory  InheritSampleTime=on  LinearizeAsDelay=on
  Vn-Vb : Sum  Inputs=+-
  PWM : Outport
  wires:
  Ipv/1 -> I Filter/1
  If DeltaP*DeltaV<0/1 -> Switch1/3
  Pn/1 -> Pn-Pb/1
  V Filter/1 -> Vn-Vb/1, Vb/1, Pn/1
  Ib/1 -> Pb/2
  DeltaP*DeltaV/1 -> Switch1/2
  Vb/1 -> Vn-Vb/2, Pb/1
  If DeltaP*DeltaV>0/1 -> Switch1/1
  Pn-Pb/1 -> DeltaP*DeltaV/1
  Vn-Vb/1 -> DeltaP*DeltaV/2
  I Filter/1 -> Pn/2, Ib/1
  Vpv/1 -> V Filter/1
  Pb/1 -> Pn-Pb/2
  Switch1/1 -> D State/2
  DeltaD/1 -> D State/1
  D State/1 -> Sum/1
  Sum/1 -> Saturation1/1
  Memory2/1 -> Sum/2
  Saturation1/1 -> PWM/1, Memory2/1

== system Commande/fuzzy logic/Fuel Cell Stack1 ==
  FuelFr : Inport
  AirFr : Inport  Port=2
  T : Inport  Port=3
  Controlled Voltage Source1 : powerlib/Electrical Sources/Controlled Voltage Source  Initialize=on  Source_Type=AC  Amplitude=0  Phase=0  Frequency=0  Measurements=None
  Current Measurement1 : powerlib/Measurements/Current Measurement  PhasorSimulation=off  OutputType=Complex  PSBequivalent=0
  Diode1 : powerlib/Power Electronics/Diode  Ron=FC.Rohm  Lon=0  Vf=0  IC=0  UseSnubber=off  Rs=1e4  Cs=inf  Measurements=off
  Gain1 : Gain  Gain=0.01
  Gain3 : Gain  Gain=0.01
  Model : Subsystem  AncestorBlock=sps_lib/Sources/Fuel Cell Stack/Model  Variant=on  VariantControlMode=label  LabelModeActiveChoice=Continuous/Detailed
      settings: AttributesFormatString=%<BlockChoice>
  PAir : Constant  Value=FC.PAir
  Pfuel : Constant  Value=FC.Pf
  x_H2 : Constant  Value=FC.x*100
  y_O2 : Constant  Value=FC.y*100
  + : PMIOPort  Tag=PMCPort  Side=Right
  - : PMIOPort  Tag=PMCPort  Port=2  Side=Right
  m : Outport  VectorParamsAs1DForOutWhenUnconnected=off
  wires:
  PAir/1 -> Model/8(PAir)
  Pfuel/1 -> Model/7(Pf)
  T/1 -> Model/2(Op Temp)
  Model/1(Voltage) -> Controlled Voltage Source1/1
  Current Measurement1/1 -> Model/1(Current)
  Model/2(m) -> m/1
  FuelFr/1 -> Model/3(H2)
  x_H2/1 -> Gain1/1
  AirFr/1 -> Model/5(Air)
  y_O2/1 -> Gain3/1
  Gain1/1 -> Model/4(x_H2)
  Gain3/1 -> Model/6(y_O2)
  connections:
  Current Measurement1/LConn1 -- Controlled Voltage Source1/RConn1
  Current Measurement1/RConn1 -- Diode1/LConn1
  -/RConn1 -- Controlled Voltage Source1/LConn1
  Diode1/RConn1 -- +/RConn1

== system Commande/fuzzy logic/Fuzzy Controller ==
  note: DE
  Vin : Inport
  P : Inport  Port=2
  Add : Sum
  DE : Sum  Inputs=+-
  E : Product  Inputs=/*
  Fuzzy Logic Controller with Ruleviewer : fuzblock/Fuzzy Logic  Controller  with Ruleviewer  fismatrix=twnty_five_rules_2  Ts=0.1
  Gain1 : Gain
  Memory1 : Memory  InheritSampleTime=on
  Memory2 : Memory  InheritSampleTime=on
  Memory3 : Memory
  Memory4 : Memory  InheritSampleTime=on
  Mux : Mux  Inputs=2
  Saturation : Saturate  UpperLimit=0.9  LowerLimit=0.1
  Zero-Order Hold : ZeroOrderHold  SampleTime=-1
  Zero-Order Hold1 : ZeroOrderHold  SampleTime=-1
  dP : Sum  Inputs=|+-
  dV : Sum  Inputs=-+
  D : Outport
  wires:
  DE/1 -> Mux/2  "DE"
  Fuzzy Logic Controller with Ruleviewer/1 -> Gain1/1  "DeltaD_Pur"
  Zero-Order Hold/1 -> dP/2, Memory1/1
  dV/1 -> E/1
  dP/1 -> E/2
  E/1 -> DE/1, Memory2/1, Mux/1  "E"
  Mux/1 -> Fuzzy Logic Controller with Ruleviewer/1
  Memory4/1 -> dV/1
  Memory1/1 -> dP/1
  Zero-Order Hold1/1 -> Memory4/1, dV/2
  Gain1/1 -> Add/1  "DeltaD"
  Memory3/1 -> Add/2
  Saturation/1 -> D/1, Memory3/1  "D"
  Memory2/1 -> DE/2
  Add/1 -> Saturation/1
  Vin/1 -> Zero-Order Hold1/1
  P/1 -> Zero-Order Hold/1

== system Commande/fuzzy logic/Fuzzy Controller2 ==
  note: DE
  Vin : Inport
  P : Inport  Port=2
  Add : Sum
  DE : Sum  Inputs=-+
  E : Product  Inputs=/*
  Fuzzy Logic Controller with Ruleviewer : fuzblock/Fuzzy Logic  Controller  with Ruleviewer  fismatrix=twnty_five_rules_5  Ts=1
  Gain1 : Gain
  Memory1 : Memory  InheritSampleTime=on
  Memory2 : Memory  InheritSampleTime=on
  Memory3 : Memory
  Memory4 : Memory  InheritSampleTime=on
  Mux : Mux  Inputs=2
  Saturation : Saturate  UpperLimit=0.9  LowerLimit=0.1
  Zero-Order Hold : ZeroOrderHold  SampleTime=-1
  Zero-Order Hold1 : ZeroOrderHold  SampleTime=-1
  dP : Sum  Inputs=-+
  dV : Sum  Inputs=+-
  D : Outport
  D1 : Outport  Port=2
  wires:
  DE/1 -> Mux/2  "DE"
  Fuzzy Logic Controller with Ruleviewer/1 -> Gain1/1  "DeltaD_Pur"
  Zero-Order Hold/1 -> dP/2, Memory1/1
  dV/1 -> E/1
  dP/1 -> E/2
  E/1 -> DE/1, Memory2/1, Mux/1  "E"
  Mux/1 -> Fuzzy Logic Controller with Ruleviewer/1
  Memory4/1 -> dV/1
  Memory1/1 -> dP/1
  Zero-Order Hold1/1 -> Memory4/1, dV/2
  Gain1/1 -> Add/1  "DeltaD"
  Memory3/1 -> Add/2
  Saturation/1 -> D/1, D1/1, Memory3/1  "D"
  Memory2/1 -> DE/2
  Add/1 -> Saturation/1
  Vin/1 -> Zero-Order Hold1/1
  P/1 -> Zero-Order Hold/1

== system Commande/INC 1/Fuel Cell Stack/Model ==
  Current : Inport
  Op Temp : Inport  Port=2
  H2 : Inport  Port=3
  x_H2 : Inport  Port=4
  Air : Inport  Port=5
  y_O2 : Inport  Port=6
  Pf : Inport  Port=7
  PAir : Inport  Port=8
  Continuous/Detailed : Subsystem  VariantControl=Continuous/Detailed
  Continuous/Simplified : Subsystem  VariantControl=Continuous/Simplified
  Discrete/Detailed : Subsystem  VariantControl=Discrete/Detailed
  Discrete/Simplified : Subsystem  VariantControl=Discrete/Simplified
  Voltage : Outport  VectorParamsAs1DForOutWhenUnconnected=off
  m : Outport  Port=2  VectorParamsAs1DForOutWhenUnconnected=off

== system Commande/P&O/Fuel Cell Stack/Model ==
  Current : Inport
  Op Temp : Inport  Port=2
  H2 : Inport  Port=3
  x_H2 : Inport  Port=4
  Air : Inport  Port=5
  y_O2 : Inport  Port=6
  Pf : Inport  Port=7
  PAir : Inport  Port=8
  Continuous/Detailed : Subsystem  VariantControl=Continuous/Detailed
  Continuous/Simplified : Subsystem  VariantControl=Continuous/Simplified
  Discrete/Detailed : Subsystem  VariantControl=Discrete/Detailed
  Discrete/Simplified : Subsystem  VariantControl=Discrete/Simplified
  Voltage : Outport  VectorParamsAs1DForOutWhenUnconnected=off
  m : Outport  Port=2  VectorParamsAs1DForOutWhenUnconnected=off

== system Commande/fuzzy logic/Fuel Cell Stack1/Model ==
  Current : Inport
  Op Temp : Inport  Port=2
  H2 : Inport  Port=3
  x_H2 : Inport  Port=4
  Air : Inport  Port=5
  y_O2 : Inport  Port=6
  Pf : Inport  Port=7
  PAir : Inport  Port=8
  Continuous/Detailed : Subsystem  VariantControl=Continuous/Detailed
  Continuous/Simplified : Subsystem  VariantControl=Continuous/Simplified
  Discrete/Detailed : Subsystem  VariantControl=Discrete/Detailed
  Discrete/Simplified : Subsystem  VariantControl=Discrete/Simplified
  Voltage : Outport  VectorParamsAs1DForOutWhenUnconnected=off
  m : Outport  Port=2  VectorParamsAs1DForOutWhenUnconnected=off

== system Commande/INC 1/Fuel Cell Stack/Model/Continuous//Detailed ==
  note: Break Algebraic
      | loop
  Current : Inport
  Op Temp : Inport  Port=2
  H2 : Inport  Port=3
  x_H2 : Inport  Port=4
  Air : Inport  Port=5
  y_O2 : Inport  Port=6
  Pf : Inport  Port=7
  PAir : Inport  Port=8
  Air consumption : Fcn  Expr=60000*FC.Nc*u(1)*FC.R*FC.Tstd/(4*FC.F*FC.Pstd*u(2))
  Bus Creator1 : BusCreator  Inputs=11
  CellVoltage : Subsystem
  Constant : Constant  Value=FC.Rohm
  Fcn2 : Fcn  Expr=u(1)-FC.Rohm*u(2)
  Fcn3 : Fcn  Expr=FC.Nc*u(1)/(FC.z*FC.F*u(2))*FC.Dh0
  Fuel consumption : Fcn  Expr=60000*FC.Nc*u(1)*FC.R*FC.Tstd/(FC.z*FC.F*FC.Pstd*u(2))
  Gain1 : Gain  Gain=100
  Gain3 : Gain  Gain=100
  Mux{,1,3..4,6} (5 alike) : Mux  Inputs=2
  Product : Product  RndMeth=Zero
  Product1 : Product  Inputs=*/  RndMeth=Zero
  Product2 : Product  RndMeth=Zero
  Saturation1 : Saturate  UpperLimit=0.9999  LowerLimit=0.0001
  Saturation2 : Saturate  UpperLimit=0.9999  LowerLimit=0.0001
  Saturation3 : Saturate  UpperLimit=inf  LowerLimit=1e-6
  Saturation4 : Saturate  UpperLimit=inf  LowerLimit=1e-3
  Saturation6 : Saturate  UpperLimit=inf  LowerLimit=0.001
  Saturation7 : Saturate  UpperLimit=inf  LowerLimit=0.001
  Saturation8 : Saturate  UpperLimit=inf  LowerLimit=200
  Selector : Selector  InputPortWidth=2  IndexOptions=Index vector (dialog)  Indices=[2]  OutputSizes=1
  Transfer Fcn : TransferFcn  Denominator=[1e-6 1]
  zero avoider : Saturate  UpperLimit=inf  LowerLimit=1e-6  LinearizeAsGain=off
  zero avoider2 : Saturate  UpperLimit=inf  LowerLimit=0  LinearizeAsGain=off
  Voltage : Outport  VectorParamsAs1DForOutWhenUnconnected=off
  m : Outport  Port=2  VectorParamsAs1DForOutWhenUnconnected=off
  wires:
  [E] -> Mux/1
  CellVoltage/7(E) -> Voltage/1, [E]
  CellVoltage/5(En) -> Bus Creator1/10  "Nerst voltage En (V)"
  Saturation2/1 -> Mux6/2, CellVoltage/6(y)  "Oxidant composition"
  CellVoltage/4(i0) -> Bus Creator1/9  "Exchange current i0 (A)"
  Product2/1 -> Bus Creator1/6  "Stack consumption (lpm) [Air(Yellow); Fuel(Magenta)]"
  Gain3/1 -> Bus Creator1/3  "Stack Efficiency (%)"
  CellVoltage/1(Fr_AirFuel) -> Bus Creator1/5, Product2/1  "Flow Rate (lpm [Air(Yellow); Fuel(Magenta)]"
  Fuel consumption/1 -> Mux3/2
  Air consumption/1 -> Mux3/1
  Gain1/1 -> Bus Creator1/7  "Utilization (%) [O2(Yellow); H2(Magenta)]"
  Selector/1 -> Mux4/2
  Mux3/1 -> Bus Creator1/4  "Stack consumption (Standard lpm) [Air(Yellow); Fuel(Magenta)]"
  Saturation4/1 -> CellVoltage/5(Air)  "Air flow rate / utilization"
  Saturation3/1 -> CellVoltage/3(H2)  "Fuel flow rate / utilization"
  Bus Creator1/1 -> m/1
  Mux6/1 -> Air consumption/1
  Mux1/1 -> Fuel consumption/1
  CellVoltage/2(Uf_O2H2) -> Product2/2, Gain1/1, Selector/1
  Transfer Fcn/1 -> Mux6/1, Mux4/1, Mux/2, Bus Creator1/2, Product/2, Mux1/1, CellVoltage/1(i)  "Current"
  Saturation8/1 -> CellVoltage/2(T)  "Operating temperature"
  Saturation7/1 -> CellVoltage/8(PAir)  "Air supply pression"
  Saturation6/1 -> CellVoltage/7(Pf)  "Fuel supply pression"
  Saturation1/1 -> Mux1/2, CellVoltage/4(x)  "Fuel composition"
  Mux4/1 -> Fcn3/1
  PAir/1 -> Saturation7/1
  Pf/1 -> Saturation6/1
  zero avoider2/1 -> Product1/1
  CellVoltage/6(Eoc) -> Bus Creator1/11  "Open circuit voltage Eoc (V)"
  CellVoltage/3(A) -> Bus Creator1/8  "Slope of Tafel curve"
  Air/1 -> Saturation4/1
  Mux/1 -> Fcn2/1
  Fcn2/1 -> Bus Creator1/1, Product/1  "Voltage"
  H2/1 -> Saturation3/1
  x_H2/1 -> Saturation1/1
  y_O2/1 -> Saturation2/1
  Op Temp/1 -> Saturation8/1
  Product/1 -> zero avoider2/1
  Fcn3/1 -> zero avoider/1
  Current/1 -> Transfer Fcn/1
  Product1/1 -> Gain3/1
  zero avoider/1 -> Product1/2

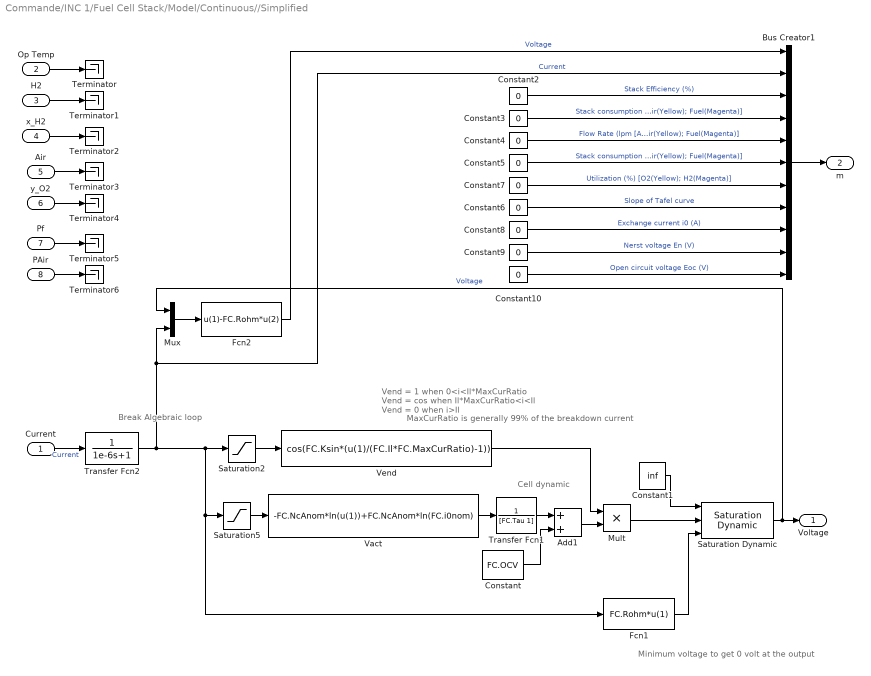
== system Commande/INC 1/Fuel Cell Stack/Model/Continuous//Simplified ==
  note: MaxCurRatio is generally 99% of the breakdown current
  note: Minimum voltage to get 0 volt at the output
  note: Cell dynamic
  note: Vend = 1 when 0<i<Il*MaxCurRatio
      | Vend = cos when Il*MaxCurRatio<i<Il
      | Vend = 0 when i>Il
  note: Break Algebraic
      | loop
  Current : Inport
  Op Temp : Inport  Port=2
  H2 : Inport  Port=3
  x_H2 : Inport  Port=4
  Air : Inport  Port=5
  y_O2 : Inport  Port=6
  Pf : Inport  Port=7
  PAir : Inport  Port=8
  Add1 : Sum
  Bus Creator1 : BusCreator  Inputs=11
  Constant : Constant  Value=FC.OCV
  Constant1 : Constant  Value=inf
  Constant{2..10} (9 alike) : Constant  Value=0
  Fcn1 : Fcn  Expr=FC.Rohm*u(1)
  Fcn2 : Fcn  Expr=u(1)-FC.Rohm*u(2)
  Mult : Product
  Mux : Mux  Inputs=2
  Saturation Dynamic : simulink/Discontinuities/Saturation Dynamic  OutMin=[]  OutMax=[]  OutDataTypeStr=Inherit: Same as second input  OutDataType=fixdt(1, 16)  OutScaling=2^-10  DoSatur=off
  Saturation2 : Saturate  UpperLimit=FC.Il  LowerLimit=FC.Il*FC.MaxCurRatio  LinearizeAsGain=off
  Saturation5 : Saturate  UpperLimit=inf  LowerLimit=FC.i0nom  LinearizeAsGain=off
  Terminator{,1..6} (7 alike) : Terminator
  Transfer Fcn1 : TransferFcn  Denominator=[FC.Tau 1]
  Transfer Fcn2 : TransferFcn  Denominator=[1e-6 1]
  Vact : Fcn  Expr=-FC.NcAnom*ln(u(1))+FC.NcAnom*ln(FC.i0nom)
  Vend : Fcn  Expr=cos(FC.Ksin*(u(1)/(FC.Il*FC.MaxCurRatio)-1))
  Voltage : Outport  VectorParamsAs1DForOutWhenUnconnected=off
  m : Outport  Port=2  VectorParamsAs1DForOutWhenUnconnected=off
  wires:
  Constant9/1 -> Bus Creator1/10  "Nerst voltage En (V)"
  Constant8/1 -> Bus Creator1/9  "Exchange current i0 (A)"
  Constant5/1 -> Bus Creator1/6  "Stack consumption (lpm) [Air(Yellow); Fuel(Magenta)]"
  Constant2/1 -> Bus Creator1/3  "Stack Efficiency (%)"
  Constant4/1 -> Bus Creator1/5  "Flow Rate (lpm [Air(Yellow); Fuel(Magenta)]"
  Constant7/1 -> Bus Creator1/7  "Utilization (%) [O2(Yellow); H2(Magenta)]"
  Constant3/1 -> Bus Creator1/4  "Stack consumption (Standard lpm) [Air(Yellow); Fuel(Magenta)]"
  Bus Creator1/1 -> m/1
  Constant10/1 -> Bus Creator1/11  "Open circuit voltage Eoc (V)"
  Constant6/1 -> Bus Creator1/8  "Slope of Tafel curve"
  Fcn2/1 -> Bus Creator1/1  "Voltage"
  PAir/1 -> Terminator6/1
  Pf/1 -> Terminator5/1
  Transfer Fcn2/1 -> Bus Creator1/2, Mux/2, Fcn1/1, Saturation5/1, Saturation2/1  "Current"
  Saturation2/1 -> Vend/1
  Vend/1 -> Mult/1
  Mult/1 -> Saturation Dynamic/2
  Add1/1 -> Mult/2
  Vact/1 -> Transfer Fcn1/1
  Fcn1/1 -> Saturation Dynamic/3
  Constant1/1 -> Saturation Dynamic/1
  Constant/1 -> Add1/2
  Transfer Fcn1/1 -> Add1/1
  Saturation Dynamic/1 -> Mux/1, Voltage/1  "Voltage"
  y_O2/1 -> Terminator4/1
  Air/1 -> Terminator3/1
  x_H2/1 -> Terminator2/1
  H2/1 -> Terminator1/1
  Op Temp/1 -> Terminator/1
  Current/1 -> Transfer Fcn2/1  "Current"
  Saturation5/1 -> Vact/1
  Mux/1 -> Fcn2/1
